simulink model "model2"  (R2021b)
settings: Solver=ode15s  StartTime=0.0  StopTime=15  FixedStep=0.013  RelTol=1e-3
model workspace (MAT data in the model file):
  U_max = 3.35
values from neighbouring files (symbols this model uses):
  B = 0.15    [compareRealToModel.m]    (also in square.m)
  goal_x = X(i)    [compareRealToModel.m]    (also in square.m)
  goal_y = Y(i)    [compareRealToModel.m]    (also in square.m)
  J = 0.0023    [compareRealToModel.m]    (also in square.m)
  k_e = 0.274    [compareRealToModel.m]    (also in square.m)
  k_m = k_e    (= 0.274)    [compareRealToModel.m]    (also in square.m)
  K_rot = 400    [compareRealToModel.m]    (also in square.m = 300)
  K_str = 100    [compareRealToModel.m]    (also in square.m = 300)
  L = 0.0047    [compareRealToModel.m]    (also in square.m)
  R = 0.025    [compareRealToModel.m]    (also in square.m)
  R_electronic = 4.73    [compareRealToModel.m]    (also in square.m)
  start_angel = simm.angel.Data(end)    [compareRealToModel.m]    (also in square.m)
  start_x = goal_x    [compareRealToModel.m]    (also in square.m)
  start_y = goal_y    [compareRealToModel.m]    (also in square.m)
settings Model: Creator=Admin  LastModifiedBy=huynh
settings SolverCC: ZeroCrossAlgorithm=Adaptive
settings DebuggingCC: IgnoredZcDiagnostic=none

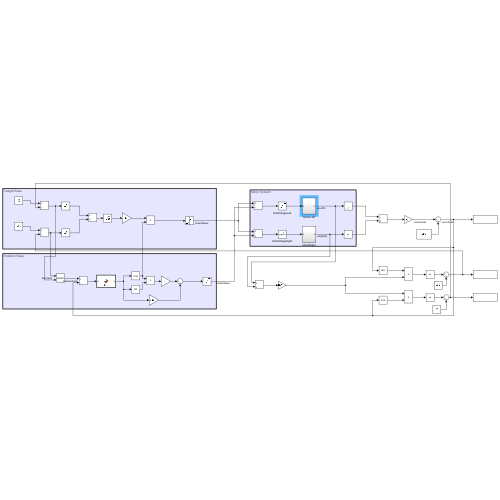
[thumbnail: Simulink's stored preview of the top-level diagram]
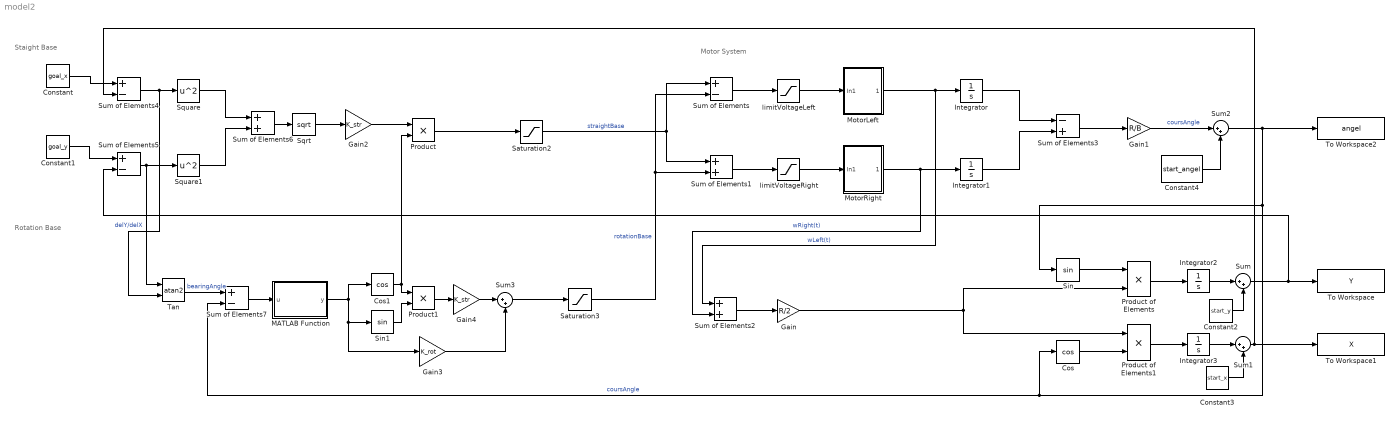
== system model2 ==
  note: Motor System
  note: Rotation Base
  note: Staight Base
  Constant : Constant  Value=goal_x
  Constant1 : Constant  Value=goal_y
  Constant2 : Constant  Value=start_y
  Constant3 : Constant  Value=start_x
  Constant4 : Constant  Value=start_angel
  Cos : Trigonometry  Operator=cos
  Cos1 : Trigonometry  Operator=cos
  Gain : Gain  Gain=R/2
  Gain1 : Gain  Gain=R/B
  Gain2 : Gain  Gain=K_str
  Gain3 : Gain  Gain=K_rot
  Gain4 : Gain  Gain=K_str
  Integrator{,1..3} (4 alike) : Integrator
  MATLAB Function : MATLAB Function  TreatAsAtomicUnit=on
  MotorLeft : Subsystem
  MotorRight : Subsystem
  Product : Product
  Product of Elements : Product  Inputs=**
  Product of Elements1 : Product  Inputs=**
  Product1 : Product
  Saturation2 : Saturate  UpperLimit=60  LowerLimit=-60
  Saturation3 : Saturate  UpperLimit=40  LowerLimit=-40
  Sin : Trigonometry
  Sin1 : Trigonometry
  Sqrt : Sqrt  SaturateOnIntegerOverflow=on
  Square : Math  Operator=square  SaturateOnIntegerOverflow=on
  Square1 : Math  Operator=square  SaturateOnIntegerOverflow=on
  Sum{,1..3} (4 alike) : Sum  Inputs=|++
  Sum of Elements{,4..5,7} (4 alike) : Sum  Inputs=+-
  Sum of Elements1 : Sum
  Sum of Elements2 : Sum
  Sum of Elements3 : Sum  Inputs=-+
  Sum of Elements6 : Sum
  Tan : Trigonometry  Operator=atan2  OutputSignalType=real
  To Workspace : ToWorkspace  VariableName=Y  SaveFormat=Timeseries  SampleTime=-1
  To Workspace1 : ToWorkspace  VariableName=X  SaveFormat=Timeseries  SampleTime=-1
  To Workspace2 : ToWorkspace  VariableName=angel  SaveFormat=Timeseries  SampleTime=-1
  limitVoltageLeft : Saturate  UpperLimit=100  LowerLimit=-100
  limitVoltageRight : Saturate  UpperLimit=100  LowerLimit=-100
  wires:
  Sum of Elements/1 -> limitVoltageLeft/1
  limitVoltageLeft/1 -> MotorLeft/1(In1)
  MotorLeft/1(Output) -> Integrator/1, Sum of Elements2/1  "wLeft(t)"
  limitVoltageRight/1 -> MotorRight/1(In1)
  Sum of Elements1/1 -> limitVoltageRight/1
  MotorRight/1(Output) -> Integrator1/1, Sum of Elements2/2  "wRight(t)"
  Sum of Elements2/1 -> Gain/1
  Integrator/1 -> Sum of Elements3/1
  Integrator1/1 -> Sum of Elements3/2
  Sum of Elements3/1 -> Gain1/1
  Sin/1 -> Product of Elements/1
  Gain/1 -> Product of Elements1/1, Product of Elements/2
  Cos/1 -> Product of Elements1/2
  Product of Elements/1 -> Integrator2/1
  Product of Elements1/1 -> Integrator3/1
  Sum2/1 -> Cos/1, Sum of Elements7/2, Sin/1, To Workspace2/1  "coursAngle"
  Integrator2/1 -> Sum/1
  Sum1/1 -> To Workspace1/1, Sum of Elements4/2
  Constant/1 -> Sum of Elements4/1
  Constant1/1 -> Sum of Elements5/1
  Sum of Elements4/1 -> Tan/2, Square/1
  Square/1 -> Sum of Elements6/1
  Square1/1 -> Sum of Elements6/2
  Sum of Elements6/1 -> Sqrt/1
  Sqrt/1 -> Gain2/1
  Sum of Elements5/1 -> Square1/1, Tan/1  "delY/delX"
  Tan/1 -> Sum of Elements7/1  "bearingAngle"
  Sum of Elements7/1 -> MATLAB Function/1(u)
  Sum3/1 -> Saturation3/1
  Saturation2/1 -> Sum of Elements/1, Sum of Elements1/1  "straightBase"
  Saturation3/1 -> Sum of Elements1/2, Sum of Elements/2  "rotationBase"
  Sum/1 -> Sum of Elements5/2, To Workspace/1
  Constant2/1 -> Sum/2
  Integrator3/1 -> Sum1/1
  Constant3/1 -> Sum1/2
  Gain1/1 -> Sum2/1  "coursAngle"
  Constant4/1 -> Sum2/2
  Gain2/1 -> Product/1
  Cos1/1 -> Product/2, Product1/1
  Product/1 -> Saturation2/1
  Sin1/1 -> Product1/2
  Product1/1 -> Gain4/1
  MATLAB Function/1(y) -> Cos1/1, Sin1/1, Gain3/1
  Gain3/1 -> Sum3/2
  Gain4/1 -> Sum3/1

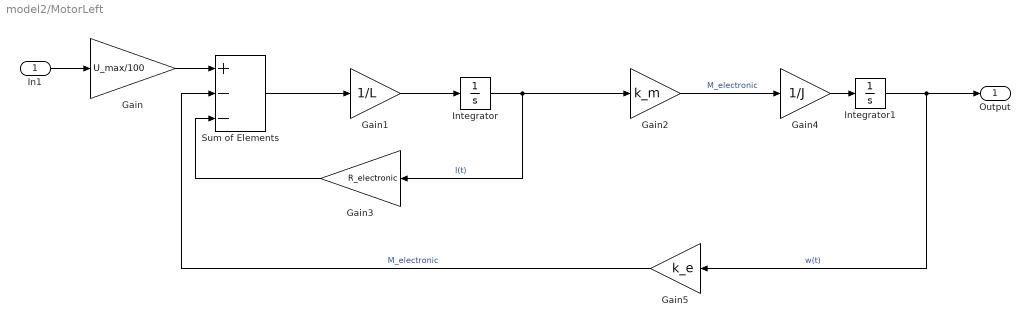
== system model2/MotorLeft ==
  In1 : Inport
  Gain : Gain  Gain=U_max/100
  Gain1 : Gain  Gain=1/L
  Gain2 : Gain  Gain=k_m
  Gain3 : Gain  Gain=R_electronic
  Gain4 : Gain  Gain=1/J
  Gain5 : Gain  Gain=k_e
  Integrator : Integrator
  Integrator1 : Integrator
  Sum of Elements : Sum  Inputs=+--
  Output : Outport
  wires:
  Gain1/1 -> Integrator/1
  Integrator/1 -> Gain3/1, Gain2/1  "I(t)"
  Gain/1 -> Sum of Elements/1
  Gain2/1 -> Gain4/1  "M_electronic"
  Sum of Elements/1 -> Gain1/1
  Gain5/1 -> Sum of Elements/2  "M_electronic"
  Gain4/1 -> Integrator1/1
  Gain3/1 -> Sum of Elements/3
  Integrator1/1 -> Gain5/1, Output/1  "w(t)"
  In1/1 -> Gain/1

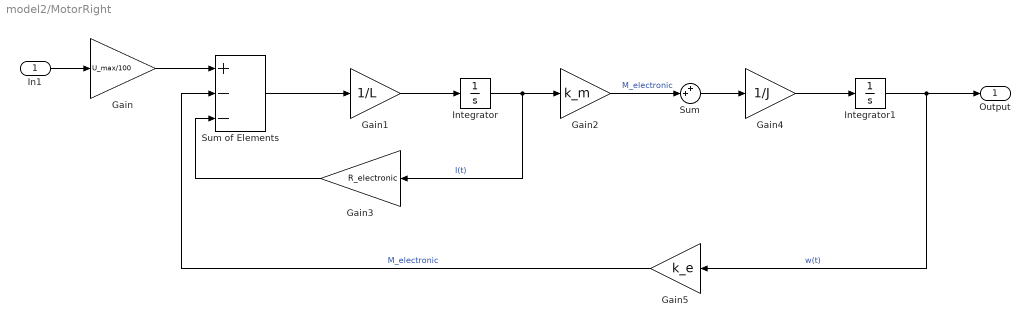
== system model2/MotorRight ==
  In1 : Inport
  Gain : Gain  Gain=U_max/100
  Gain1 : Gain  Gain=1/L
  Gain2 : Gain  Gain=k_m
  Gain3 : Gain  Gain=R_electronic
  Gain4 : Gain  Gain=1/J
  Gain5 : Gain  Gain=k_e
  Integrator : Integrator
  Integrator1 : Integrator
  Sum : Sum  Inputs=++|
  Sum of Elements : Sum  Inputs=+--
  Output : Outport
  wires:
  Gain1/1 -> Integrator/1
  Integrator/1 -> Gain3/1, Gain2/1  "I(t)"
  Sum/1 -> Gain4/1
  Gain/1 -> Sum of Elements/1
  Gain2/1 -> Sum/2  "M_electronic"
  Sum of Elements/1 -> Gain1/1
  Gain5/1 -> Sum of Elements/2  "M_electronic"
  Gain4/1 -> Integrator1/1
  Gain3/1 -> Sum of Elements/3
  Integrator1/1 -> Output/1, Gain5/1  "w(t)"
  In1/1 -> Gain/1

== matlab function model2/MATLAB Function ==
  data: u input; y output
function y = fcn(u)
if abs(u) > pi
    y = u - sign(u)*2*pi;
else
    y = u;    
end
